simulink model "Ex2_2"  (R2016b)
settings: Solver=VariableStepAuto  StartTime=0.0  StopTime=10  RelTol=1e-3
values from neighbouring files (symbols this model uses):
  D = 1    [Ex2_2_init.m]
  g = 9.81    [Ex2_2_init.m]
  k = 100    [Ex2_2_init.m]    (also in Ex2_5_init.m = 5000)
  m = 1.5    [Ex2_2_init.m]
  Zs = 0.2    [Ex2_2_init.m]
settings Model: Creator=Niels  LastModifiedBy=Niels

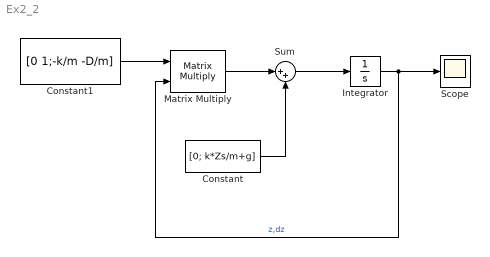
== system Ex2_2 ==
  Constant : Constant  Value=[0; k*Zs/m+g]
  Constant1 : Constant  Value=[0 1;-k/m -D/m]
  Integrator : Integrator  InitialCondition=[0.1; 0]
  Matrix Multiply : Product  Multiplication=Matrix(*)
  Scope : Scope
  Sum : Sum  Inputs=|++
  wires:
  Matrix Multiply/1 -> Sum/1
  Sum/1 -> Integrator/1
  Constant/1 -> Sum/2
  Constant1/1 -> Matrix Multiply/1
  Integrator/1 -> Matrix Multiply/2, Scope/1  "z,dz"
